simulink model "bitwise"  (R2021a)
settings: Solver=FixedStepDiscrete  StartTime=0.0  StopTime=10.0  RelTol=1e-3  EnableMultiTasking=on
libraries: simulink x6
settings Model: Creator=iT-User  LastModifiedBy=iT-User
settings DataIOCC: ReturnWorkspaceOutputs=off
settings OptimizationCC: DefaultParameterBehavior=Inlined  InlineInvariantSignals=on  EnableMemcpy=off  LifeSpan=1  EfficientTunableParamExpr=on
settings DebuggingCC: UnderspecifiedInitializationDetection=Classic  MergeDetectMultiDrivingBlocksExec=none  SFMachineParentedDataDiag=warning  ArithmeticOperatorsInVariantConditions=warning
settings ModelReferenceCC: PropagateSignalLabelsOutOfModel=off
settings SFSimCC: MATLABDynamicMemAlloc=off  CustomCodeUndefinedFunction=UseInterfaceOnly
settings RTWCC: SystemTargetFile=ert.tlc  GenCodeOnly=on  TemplateMakefile=ert_default_tmf  GenerateReport=on  IncludeHyperlinkInReport=on  LaunchReport=on  GenerateTraceInfo=on  GenerateTraceReport=on  GenerateTraceReportSl=on  GenerateTraceReportSf=on  GenerateTraceReportEml=on
settings CodeAppCC: ForceParamTrailComments=on  IgnoreCustomStorageClasses=off  OperatorAnnotations=on  SimulinkDataObjDesc=on  SFDataObjDesc=on  MATLABFcnDesc=on  InsertBlockDesc=on  StateflowObjectComments=on  MATLABSourceComments=on
settings ERTTargetCC: MultiwordLength=2048  GenerateSampleERTMain=on  InlinedParameterPlacement=NonHierarchical  ERTCustomFileTemplate=example_file_process.tlc

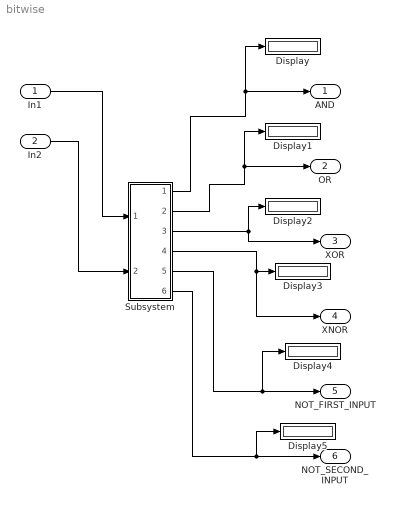
== system bitwise ==
  In1 : Inport  OutDataTypeStr=uint32
  In2 : Inport  Port=2  OutDataTypeStr=uint32
  Display{,1..5} (6 alike) : Display
  Subsystem : Subsystem
  AND : Outport  OutDataTypeStr=uint32
  OR : Outport  Port=2  OutDataTypeStr=uint32
  XOR : Outport  Port=3  OutDataTypeStr=uint32
  XNOR : Outport  Port=4  OutDataTypeStr=uint32
  NOT_FIRST_INPUT : Outport  Port=5  OutDataTypeStr=uint32
  NOT_SECOND_INPUT : Outport  Port=6  OutDataTypeStr=uint32
  wires:
  Subsystem/5(Out5) -> Display4/1, NOT_FIRST_INPUT/1
  Subsystem/3(Out3) -> XOR/1, Display2/1
  Subsystem/4(Out4) -> XNOR/1, Display3/1
  Subsystem/2(Out2) -> Display1/1, OR/1
  Subsystem/6(Out6) -> Display5/1, NOT_SECOND_INPUT/1
  Subsystem/1(Out1) -> Display/1, AND/1
  In1/1 -> Subsystem/1(In1)
  In2/1 -> Subsystem/2(In2)

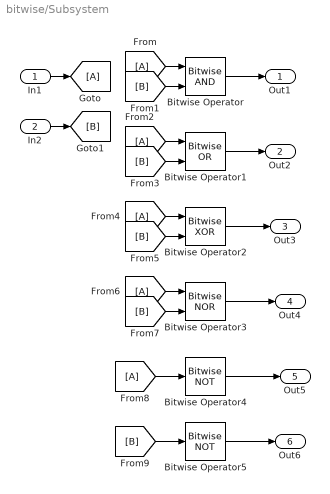
== system bitwise/Subsystem ==
  In1 : Inport
  In2 : Inport  Port=2
  Bitwise Operator : simulink/Logic and Bit Operations/Bitwise Operator  logicop=AND  UseBitMask=off  NumInputPorts=2  BitMask=bin2dec('11011001')  BitMaskRealWorld=Stored Integer
  Bitwise Operator1 : simulink/Logic and Bit Operations/Bitwise Operator  logicop=OR  UseBitMask=off  NumInputPorts=2  BitMask=bin2dec('11011001')  BitMaskRealWorld=Stored Integer
  Bitwise Operator2 : simulink/Logic and Bit Operations/Bitwise Operator  logicop=XOR  UseBitMask=off  NumInputPorts=2  BitMask=bin2dec('11011001')  BitMaskRealWorld=Stored Integer
  Bitwise Operator3 : simulink/Logic and Bit Operations/Bitwise Operator  logicop=NOR  UseBitMask=off  NumInputPorts=2  BitMask=bin2dec('11011001')  BitMaskRealWorld=Stored Integer
  Bitwise Operator4 : simulink/Logic and Bit Operations/Bitwise Operator  logicop=NOT  UseBitMask=off  BitMask=bin2dec('11011001')  BitMaskRealWorld=Stored Integer
  Bitwise Operator5 : simulink/Logic and Bit Operations/Bitwise Operator  logicop=NOT  UseBitMask=off  BitMask=bin2dec('11011001')  BitMaskRealWorld=Stored Integer
  Out1 : Outport
  Out2 : Outport  Port=2
  Out3 : Outport  Port=3
  Out4 : Outport  Port=4
  Out5 : Outport  Port=5
  Out6 : Outport  Port=6
  wires:
  [B] -> Bitwise Operator/2
  [A] -> Bitwise Operator1/1
  [A] -> Bitwise Operator/1
  [B] -> Bitwise Operator2/2
  [A] -> Bitwise Operator3/1
  [A] -> Bitwise Operator4/1
  [B] -> Bitwise Operator1/2
  [B] -> Bitwise Operator3/2
  [A] -> Bitwise Operator2/1
  Bitwise Operator1/1 -> Out2/1
  [B] -> Bitwise Operator5/1
  Bitwise Operator4/1 -> Out5/1
  In2/1 -> [B]
  In1/1 -> [A]
  Bitwise Operator3/1 -> Out4/1
  Bitwise Operator5/1 -> Out6/1
  Bitwise Operator/1 -> Out1/1
  Bitwise Operator2/1 -> Out3/1
